simulink model "car_PID_parallal"  (R2019a)
settings: Solver=VariableStepAuto  StartTime=0.0  StopTime=100  RelTol=1e-3
values from neighbouring files (symbols this model uses):
  a = [0.328350063485 -0.504393436497 -18.7824329195 1.02511531984 -53.4041424252]    [a.mat]    (also in a1.mat = [-0.685212439995 -0.585400025674 -24.4194734415 0.9475851353; a2.mat = [-1.28043820376 -0.621828624231 -54.7528450797 1.71837449641; system_id.m = pinv(G1'*G1)*G1'*E)
  b = [6.12465019513 -5.20663579301 6.03715613869 77.417940964 10.1407211952]    [b.mat]    (also in b1.mat = [34.2019090673 -33.7070179637 52.7248095782 336.319136551 44; b2.mat = [16.939936533 -14.6014953721 67.1462611587 436.465012222 564; system_id.m = pinv(G2'*G2)*G2'*E)
undefined symbols (not defined in the file or in its folder): DiscIntNeverNeededParam
libraries: simulink x2
settings Model: Creator=ray  LastModifiedBy=ASUS
settings DebuggingCC: AlgebraicLoopMsg=none

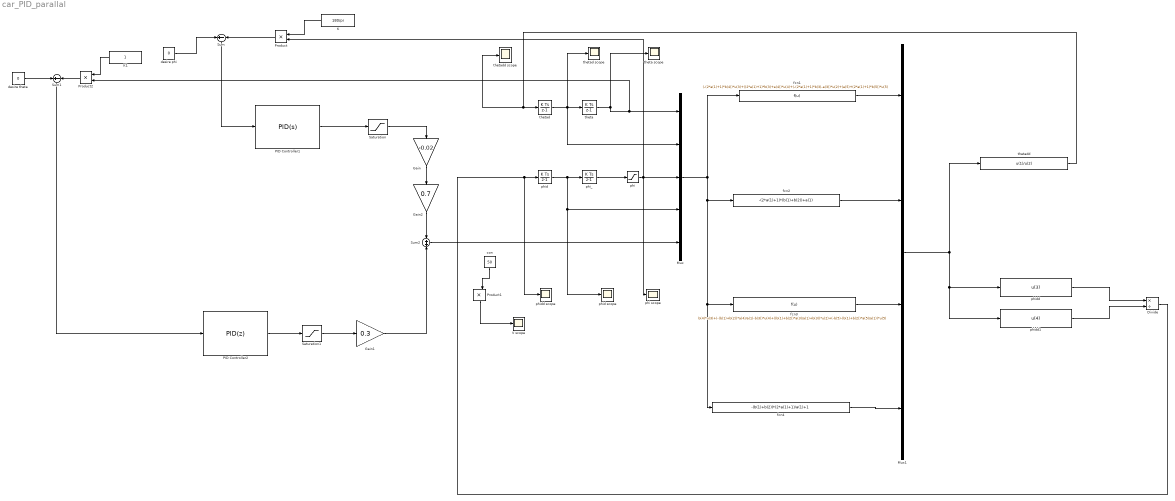
== system car_PID_parallal ==
  Divide : Product  Inputs=*/
  Gain : Gain  Gain=-0.02
  Gain1 : Gain  Gain=0.3
  Gain2 : Gain  Gain=0.7
  "K " : Constant  Value=180/pi  SampleTime=0.01
  K1 : Constant  SampleTime=0.01
  Mux : Mux  Inputs=5
  Mux1 : Mux
  PID Controller1 : simulink/Continuous/PID Controller  Controller=PID  Form=Parallel  TimeDomain=Continuous-time  SampleTime=0.001  IntegratorMethod=Forward Euler  FilterMethod=Forward Euler  ControllerParametersSource=internal  P=3  I=80  D=0  UseFilter=on  N=100  TunerSelectOption=Transfer Function Based (PID Tuner App)  InitialConditionSource=internal  InitialConditionForIntegrator=0  InitialConditionForFilter=0  DifferentiatorICPrevScaledInput=0  ExternalReset=none  TrackingMode=off  Kt=1  LimitOutput=off  UpperSaturationLimit=inf  LowerSaturationLimit=-inf  LinearizeAsGain=on  AntiWindupMode=none  Kb=1  POutMin=[]  POutMax=[]  IOutMin=[]  IOutMax=[]  DOutMin=[]  DOutMax=[]  NOutMin=[]  NOutMax=[]  SumOutMin=[]  SumOutMax=[]  SaturationOutMin=[]  SaturationOutMax=[]  PParamMin=[]  PParamMax=[]  IParamMin=[]  IParamMax=[]  DParamMin=[]  DParamMax=[]  NParamMin=[]  NParamMax=[]  KbParamMin=[]  KbParamMax=[]  KtParamMin=[]  KtParamMax=[]  KbOutMin=[]  KbOutMax=[]  KtOutMin=[]  KtOutMax=[]  IntegratorOutMin=[]  IntegratorOutMax=[]  FilterOutMin=[]  FilterOutMax=[]  SumI1OutMin=[]  SumI1OutMax=[]  SumI2OutMin=[]  SumI2OutMax=[]  SumI3OutMin=[]  SumI3OutMax=[]  SumI4OutMin=[]  SumI4OutMax=[]  SumDOutMin=[]  SumDOutMax=[]  DifferentiatorOutMin=[]  DifferentiatorOutMax=[]  FilterDiffOutCoefMin=[]  FilterDiffOutCoefMax=[]  ReciprocalOutMin=[]  ReciprocalOutMax=[]  SumDenOutMin=[]  SumDenOutMax=[]  SumNumOutMin=[]  SumNumOutMax=[]  DivideOutMin=[]  DivideOutMax=[]  IntegratorContinuousStateAttributes=''  IntegratorStateMustResolveToSignalObject=off  IntegratorRTWStateStorageClass=Auto  FilterContinuousStateAttributes=''  FilterStateMustResolveToSignalObject=off  FilterRTWStateStorageClass=Auto  ParallelPVariant=InternalParameters  IdealPVariant=Disabled  IVariant=InternalParameters  DVariant=InternalParameters  IntegratorVariant=Continuous  SatVariant=Disabled  AWVariant=Passthrough  PCopyVariant=Disabled  TRVariant=Disabled  FdbkBlocksVariant=Forward  IdealPFdbkVariant=Disabled  SatFdbkVariant=Disabled  DerivativeFilterVariant=ContFilter  NVariant=InternalParameters  NCopyVariant=Disabled  FilterICVariant=InternalICsFilter  IntegratorICVariant=InternalICs  ExternalResetVariant=Disabled  TRSumVariant=Passthrough  SumFdbkVariant=Disabled  SumVariant=Sum_PID
  PID Controller2 : simulink/Continuous/PID Controller  Controller=PID  Form=Parallel  TimeDomain=Discrete-time  SampleTime=0.001  IntegratorMethod=Forward Euler  FilterMethod=Forward Euler  ControllerParametersSource=internal  P=9  I=200  D=0.05  UseFilter=on  N=100  TunerSelectOption=Transfer Function Based (PID Tuner App)  InitialConditionSource=internal  InitialConditionForIntegrator=0  InitialConditionForFilter=0  DifferentiatorICPrevScaledInput=0  ExternalReset=none  TrackingMode=off  Kt=1  LimitOutput=off  UpperSaturationLimit=inf  LowerSaturationLimit=-inf  LinearizeAsGain=on  AntiWindupMode=none  Kb=1  POutMin=[]  POutMax=[]  IOutMin=[]  IOutMax=[]  DOutMin=[]  DOutMax=[]  NOutMin=[]  NOutMax=[]  SumOutMin=[]  SumOutMax=[]  SaturationOutMin=[]  SaturationOutMax=[]  PParamMin=[]  PParamMax=[]  IParamMin=[]  IParamMax=[]  DParamMin=[]  DParamMax=[]  NParamMin=[]  NParamMax=[]  KbParamMin=[]  KbParamMax=[]  KtParamMin=[]  KtParamMax=[]  KbOutMin=[]  KbOutMax=[]  KtOutMin=[]  KtOutMax=[]  IntegratorOutMin=[]  IntegratorOutMax=[]  FilterOutMin=[]  FilterOutMax=[]  SumI1OutMin=[]  SumI1OutMax=[]  SumI2OutMin=[]  SumI2OutMax=[]  SumI3OutMin=[]  SumI3OutMax=[]  SumI4OutMin=[]  SumI4OutMax=[]  SumDOutMin=[]  SumDOutMax=[]  DifferentiatorOutMin=[]  DifferentiatorOutMax=[]  FilterDiffOutCoefMin=[]  FilterDiffOutCoefMax=[]  ReciprocalOutMin=[]  ReciprocalOutMax=[]  SumDenOutMin=[]  SumDenOutMax=[]  SumNumOutMin=[]  SumNumOutMax=[]  DivideOutMin=[]  DivideOutMax=[]  IntegratorContinuousStateAttributes=''  IntegratorStateMustResolveToSignalObject=off  IntegratorRTWStateStorageClass=Auto  FilterContinuousStateAttributes=''  FilterStateMustResolveToSignalObject=off  FilterRTWStateStorageClass=Auto  ParallelPVariant=InternalParameters  IdealPVariant=Disabled  IVariant=InternalParameters  DVariant=InternalParameters  IntegratorVariant=Discrete  SatVariant=Disabled  AWVariant=Passthrough  PCopyVariant=Disabled  TRVariant=Disabled  FdbkBlocksVariant=Forward  IdealPFdbkVariant=Disabled  SatFdbkVariant=Disabled  DerivativeFilterVariant=ForwardEulerFilter  NVariant=InternalParameters  NCopyVariant=Disabled  FilterICVariant=InternalICsFilter  IntegratorICVariant=InternalICs  ExternalResetVariant=Disabled  TRSumVariant=Passthrough  SumFdbkVariant=Disabled  SumVariant=Sum_PID
  Product : Product
  Product1 : Product
  Product2 : Product
  Saturation : Saturate  UpperLimit=100  LowerLimit=-100
  Saturation1 : Saturate  UpperLimit=0.1  LowerLimit=-0.1
  Sum : Sum  Inputs=+-
  Sum1 : Sum  Inputs=+-
  Sum2 : Sum
  "V scope " : Scope
  "con " : Constant  Value=50  SampleTime=0.01
  "desire phi " : Constant  Value=0  SampleTime=0.001
  "desire theta " : Constant  Value=0  SampleTime=0.001
  fcn1 : Fcn  Expr=(-(2*a(1)+1)*b(4))*u(3)+((2*a(1)+1)*b(3)+a(4))*u(4)+(-(2*a(1)+1)*b(3)-a(3))*u(2)+(a(5)+(2*a(1)+1)*b(5))*u(5)
  fcn2 : Fcn  Expr=-(2*a(1)+1)*(b(1)+b(2))+a(1)
  fcn3 : Fcn  Expr=b(4)*u(3)+(-(b(1)+b(2))*a(4)/a(1)-b(3))*u(4)+((b(1)+b(2))*a(3)/a(1)+b(3))*u(2)+(-b(5)-(b(1)+b(2))*a(5)/a(1))*u(5)
  fcn4 : Fcn  Expr=-(b(1)+b(2))*(2*a(1)+1)/a(1)+1
  phi : Saturate  UpperLimit=1.6  LowerLimit=-1.6
  "phi scope " : Scope
  phi_ : DiscreteIntegrator  InitialCondition=0.01  SampleTime=0.001  ICPrevOutput=DiscIntNeverNeededParam  ICPrevScaledInput=DiscIntNeverNeededParam
  phid : DiscreteIntegrator  SampleTime=0.001  ICPrevOutput=DiscIntNeverNeededParam  ICPrevScaledInput=DiscIntNeverNeededParam
  "phid scope " : Scope
  phidd : Fcn  Expr=u(3)
  "phidd scope " : Scope
  phidd1 : Fcn  Expr=u(4)
  theta : DiscreteIntegrator  SampleTime=0.001  ICPrevOutput=DiscIntNeverNeededParam  ICPrevScaledInput=DiscIntNeverNeededParam
  theta scope : Scope
  thetad : DiscreteIntegrator  SampleTime=0.001  ICPrevOutput=DiscIntNeverNeededParam  ICPrevScaledInput=DiscIntNeverNeededParam
  "thetad scope " : Scope
  thetadd : Fcn  Expr=u(1)/u(2)
  "thetadd scope " : Scope
  wires:
  phid/1 -> Mux/4, "phid scope "/1, phi_/1
  phi_/1 -> phi/1
  phi/1 -> Product/2, Mux/3, "phi scope "/1
  fcn4/1 -> Mux1/4
  fcn3/1 -> Mux1/3
  fcn2/1 -> Mux1/2
  fcn1/1 -> Mux1/1
  theta/1 -> theta scope/1, Product2/2, Mux/1
  Mux1/1 -> thetadd/1, phidd1/1, phidd/1
  Mux/1 -> fcn2/1, fcn3/1, fcn4/1, fcn1/1
  thetad/1 -> "thetad scope "/1, Mux/2, theta/1
  thetadd/1 -> "thetadd scope "/1, thetad/1
  phidd/1 -> Divide/1
  phidd1/1 -> Divide/2
  Divide/1 -> "phidd scope "/1, phid/1
  PID Controller1/1 -> Saturation/1
  Saturation/1 -> Gain/1
  "desire phi "/1 -> Sum/1
  "K "/1 -> Product/1
  Product/1 -> Sum/2
  Product1/1 -> "V scope "/1
  "con "/1 -> Product1/2
  Sum/1 -> PID Controller1/1
  "desire theta "/1 -> Sum1/1
  Sum1/1 -> PID Controller2/1
  PID Controller2/1 -> Saturation1/1
  Product2/1 -> Sum1/2
  K1/1 -> Product2/1
  Gain1/1 -> Sum2/2
  Sum2/1 -> Mux/5
  Gain/1 -> Gain2/1
  Gain2/1 -> Sum2/1
  Saturation1/1 -> Gain1/1
